simulink model "IDC_OS"  (R2023b)
settings: Solver=FixedStepAuto  StartTime=0.0  StopTime=9  FixedStep=sampleTime  RelTol=1e-3
values from neighbouring files (symbols this model uses):
  initialguess = robot.homeConfiguration    [IDC_OS.m]
  K_D = 0*eye(n_joints)    [IDC_OS.m]
  K_P = 0*eye(n_joints)    [IDC_OS.m]
  n_joints = 6    [IDC_OS.m]
  robot = loadrobot("universalUR5")    [IDC_OS.m]
  t0 = 0    [IDC_OS.m]
  t1 = 5    [IDC_OS.m]
  t2 = 10    [IDC_OS.m]
  t3 = 100    [IDC_OS.m]
  weights = transpose([0.1, 0.1, 0.1, 1, 1, 1])    [IDC_OS.m]
  x0_pose = trvec2tform([x0(1), x0(2), x0(3)]) * eul2tform([x0(4), x0(5), x0(6)])    [IDC_OS.m]
  xd = zeros(n_joints,1)    [IDC_OS.m]
undefined symbols (not defined in the file or in its folder): x1_pose, x2_pose
libraries: robotmaniplib x8
(part 1 of 2)
settings Model: Creator=Mikael  LastModifiedBy=Mikael

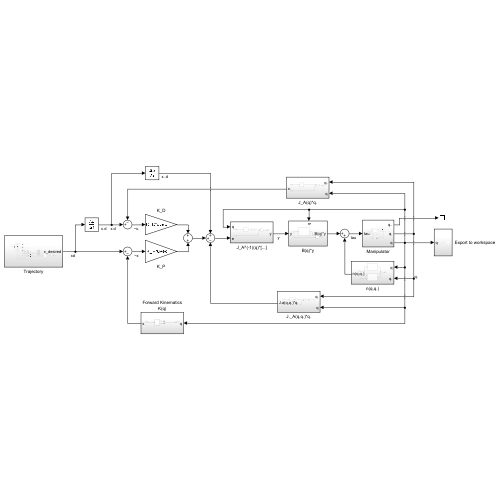
[thumbnail: Simulink's stored preview of the top-level diagram]
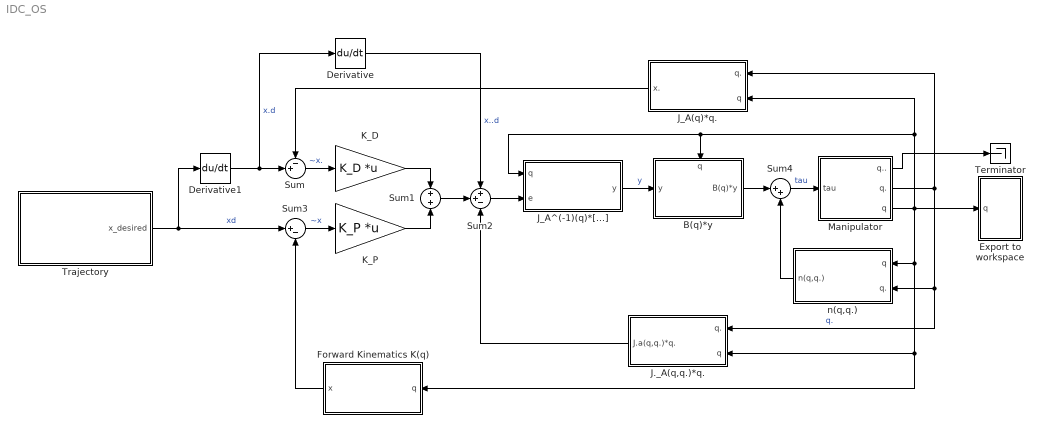
== system IDC_OS ==
  B(q)*y : Subsystem
      settings: PortSchema="{\"entries\":[{\"content\":{\"sides\":[{\"content\":{\"connectorIds\":[\"In1\"]},\"type\":\"ConnectorPlacement.EquallySpacedRectSide\",\"uuid\":\"33913df9-fd91-41b2-9bc7-1b3e33a51275\"},{\"content\":{\"connectorIds\":[\"Out1\"],\"side\":\"RIGHT\"},\"type\":\"ConnectorPlacement.EquallySpacedRectSide\",\"uuid\":\"b12fb46d-67b4-41c7-9bd3-75276d256d3b\"},{\"content\":{\"connectorIds\":[\"In2\"],\"side\":\"TOP\"},\"type\":\"ConnectorPlacement.EquallySpacedRectSide\",\"uuid\":\"ba102851-dd76-427a-8601-5d449287c868\"}]},\"type\":\"ConnectorPlacement.EquallySpacedConnector\",\"uuid\":\"a91f0b44-1456-4575-973a-6fc50432c507\"}],\"packageUris\":[\"http://schema.mathworks.com/mf0/Connector/R2020b\"],\"version\":\"1.0\"}"
  Derivative : Derivative
  Derivative1 : Derivative
  Export to workspace : Subsystem
  Forward Kinematics K(q) : Subsystem
  J._A(q,q.)*q. : Subsystem
  J_A(q)*q. : Subsystem
  J_A^(-1)(q)*[...] : Subsystem
  K_D : Gain  Gain=K_D  Multiplication=Matrix(K*u) (u vector)
  K_P : Gain  Gain=K_P  Multiplication=Matrix(K*u) (u vector)
  Manipulator : Subsystem
  Sum : Sum  Inputs=-+|
  Sum1 : Sum
  Sum2 : Sum  Inputs=++-
  Sum3 : Sum  Inputs=|+-
  Sum4 : Sum  Inputs=|++
  Terminator : Terminator
  Trajectory : Subsystem
  n(q,q.) : Subsystem
  wires:
  Manipulator/3(q) -> B(q)*y/2(q), J_A^(-1)(q)*[...]/1(q), J_A(q)*q./2(q), Export to workspace/1(q), J._A(q,q.)*q./2(q), Forward Kinematics K(q)/1(q), n(q,q.)/1(q)
  Manipulator/2(q.) -> J_A(q)*q./1(q.), J._A(q,q.)*q./1(q.), n(q,q.)/2(q.)  "q."
  Sum4/1 -> Manipulator/1(tau)  "tau"
  J_A(q)*q./1(x.) -> Sum/1
  Sum/1 -> K_D/1  "~x."
  Sum3/1 -> K_P/1  "~x"
  K_D/1 -> Sum1/1
  K_P/1 -> Sum1/2
  Sum2/1 -> J_A^(-1)(q)*[...]/2(e)
  Sum1/1 -> Sum2/2
  B(q)*y/1(B(q)*y) -> Sum4/1
  J_A^(-1)(q)*[...]/1(y) -> B(q)*y/1(y)  "y"
  n(q,q.)/1(n(q,q.)) -> Sum4/2
  J._A(q,q.)*q./1(J.a(q,q.)*q.) -> Sum2/3
  Forward Kinematics K(q)/1(x) -> Sum3/2
  Trajectory/1(x_desired) -> Sum3/1, Derivative1/1  "xd"
  Derivative1/1 -> Sum/2, Derivative/1  "x.d"
  Derivative/1 -> Sum2/1  "x..d"
  Manipulator/1(q..) -> Terminator/1

== system IDC_OS/B(q)*y ==
  y : Inport
  q : Inport  Port=2
  B(q) : robotmaniplib/Joint Space Mass Matrix  RigidBodyTree=robot  SimulateUsing=Code generation
  Matrix Multiply : Product  Multiplication=Matrix(*)
  B(q)*y : Outport
  wires:
  y/1 -> Matrix Multiply/2
  q/1 -> B(q)/1
  Matrix Multiply/1 -> B(q)*y/1
  B(q)/1 -> Matrix Multiply/1

== system IDC_OS/Export to workspace ==
  note: Export to workspace as:
      | - Array
      | - Save 2-D Signal as 3-D signal
      | (concatenated along the third dimension)
  q : Inport
  Signal Specification : SignalSpecification  Dimensions=[6,1]
  To Workspace2 : ToWorkspace  VariableName=q  SampleTime=-1
  wires:
  q/1 -> Signal Specification/1
  Signal Specification/1 -> To Workspace2/1

== system IDC_OS/Forward Kinematics K(q) ==
  q : Inport
  Direct Kinematics : Subsystem
  Mux : Mux  Inputs=2
  x : Outport
  wires:
  q/1 -> Direct Kinematics/1(q)
  Mux/1 -> x/1
  Direct Kinematics/1(position) -> Mux/1
  Direct Kinematics/2(orientation) -> Mux/2

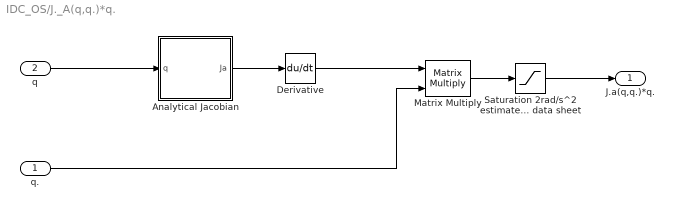
== system IDC_OS/J._A(q,q.)*q. ==
  q. : Inport
  q : Inport  Port=2
  Analytical Jacobian : Subsystem
  Derivative : Derivative
  Matrix Multiply : Product  Multiplication=Matrix(*)
  Saturation 2rad/s^2 estimated based on data sheet : Saturate  UpperLimit=2  LowerLimit=-2
  J.a(q,q.)*q. : Outport
  wires:
  q/1 -> Analytical Jacobian/1(q)
  q./1 -> Matrix Multiply/2
  Analytical Jacobian/1(Ja) -> Derivative/1
  Derivative/1 -> Matrix Multiply/1
  Matrix Multiply/1 -> Saturation 2rad/s^2 estimated based on data sheet/1
  Saturation 2rad/s^2 estimated based on data sheet/1 -> J.a(q,q.)*q./1

== system IDC_OS/J_A(q)*q. ==
  q. : Inport
  q : Inport  Port=2
  Analytical Jacobian : Subsystem
  Matrix Multiply : Product  Multiplication=Matrix(*)
  x. : Outport
  wires:
  q/1 -> Analytical Jacobian/1(q)
  q./1 -> Matrix Multiply/2
  Analytical Jacobian/1(Ja) -> Matrix Multiply/1
  Matrix Multiply/1 -> x./1

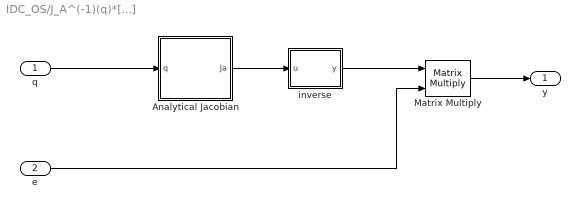
== system IDC_OS/J_A^(-1)(q)*[...] ==
  q : Inport
  e : Inport  Port=2
  Analytical Jacobian : Subsystem
  Matrix Multiply : Product  Multiplication=Matrix(*)
  inverse : MATLAB Function  TreatAsAtomicUnit=on
  y : Outport
  wires:
  q/1 -> Analytical Jacobian/1(q)
  e/1 -> Matrix Multiply/2
  inverse/1(y) -> Matrix Multiply/1
  Analytical Jacobian/1(Ja) -> inverse/1(u)
  Matrix Multiply/1 -> y/1

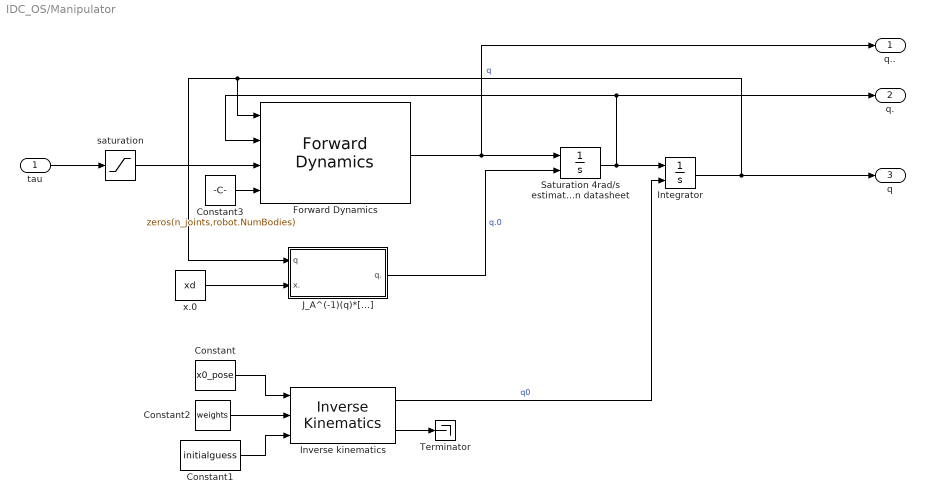
== system IDC_OS/Manipulator ==
  tau : Inport
  Constant : Constant  Value=x0_pose
  Constant1 : Constant  Value=initialguess
  Constant2 : Constant  Value=weights
  Constant3 : Constant  Value=zeros(n_joints,robot.NumBodies)
  Forward Dynamics : robotmaniplib/Forward Dynamics  RigidBodyTree=robot  SimulateUsing=Code generation
  Integrator : Integrator  InitialConditionSource=external
  Inverse kinematics : robotmaniplib/Inverse Kinematics  RigidBodyTree=robot  EndEffector=tool0  ShowInfo=on  SolverName=BFGS Gradient Projection  EnforceJointLimits=on  MaxIterations=1500  MaxTime=10  GradientTolerance=1e-7  SolutionTolerance=1e-6  StepTolerance=1e-14  ErrorChangeTolerance=1e-12  UseErrorDamping=on  DampingBias=0.0025  SimulateUsing=Code generation
  J_A^(-1)(q)*[...] : Subsystem
  Saturation 4rad/s estimated based on datasheet : Integrator  InitialConditionSource=external  LimitOutput=on  UpperSaturationLimit=4  LowerSaturationLimit=-4
  Terminator : Terminator
  saturation : Saturate  UpperLimit=inf  LowerLimit=-inf
  x.0 : Constant  Value=xd
  q.. : Outport
  q. : Outport  Port=2
  q : Outport  Port=3
  wires:
  Integrator/1 -> Forward Dynamics/1, J_A^(-1)(q)*[...]/1(q), q/1  "q"
  tau/1 -> saturation/1
  Inverse kinematics/1 -> Integrator/2  "q0"
  Constant/1 -> Inverse kinematics/1
  Constant2/1 -> Inverse kinematics/2
  Constant1/1 -> Inverse kinematics/3
  Saturation 4rad/s estimated based on datasheet/1 -> q./1, Forward Dynamics/2, Integrator/1
  saturation/1 -> Forward Dynamics/3
  Forward Dynamics/1 -> q../1, Saturation 4rad/s estimated based on datasheet/1
  J_A^(-1)(q)*[...]/1(q.) -> Saturation 4rad/s estimated based on datasheet/2  "q.0"
  x.0/1 -> J_A^(-1)(q)*[...]/2(x.)
  Constant3/1 -> Forward Dynamics/4
  Inverse kinematics/2 -> Terminator/1

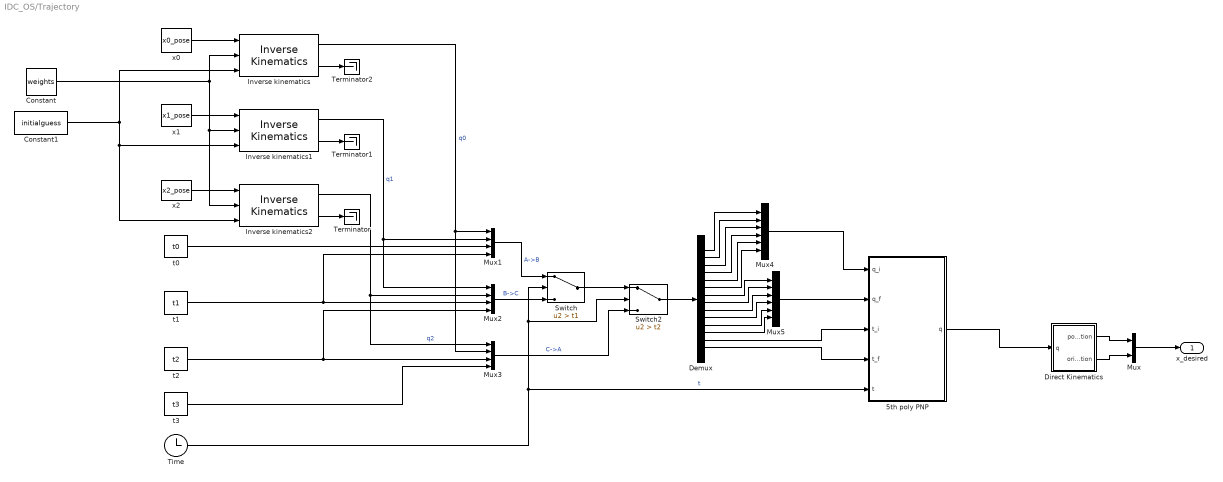
== system IDC_OS/Trajectory ==
  5th poly PNP : MATLAB Function  TreatAsAtomicUnit=on
  Constant : Constant  Value=weights
  Constant1 : Constant  Value=initialguess
  Demux : Demux  Outputs=14
  Direct Kinematics : Subsystem
  Inverse kinematics : robotmaniplib/Inverse Kinematics  RigidBodyTree=robot  EndEffector=tool0  ShowInfo=on  SolverName=BFGS Gradient Projection  EnforceJointLimits=on  MaxIterations=1500  MaxTime=10  GradientTolerance=1e-7  SolutionTolerance=1e-6  StepTolerance=1e-14  ErrorChangeTolerance=1e-12  UseErrorDamping=on  DampingBias=0.0025  SimulateUsing=Code generation
  Inverse kinematics1 : robotmaniplib/Inverse Kinematics  RigidBodyTree=robot  EndEffector=tool0  ShowInfo=on  SolverName=BFGS Gradient Projection  EnforceJointLimits=on  MaxIterations=1500  MaxTime=10  GradientTolerance=1e-7  SolutionTolerance=1e-6  StepTolerance=1e-14  ErrorChangeTolerance=1e-12  UseErrorDamping=on  DampingBias=0.0025  SimulateUsing=Code generation
  Inverse kinematics2 : robotmaniplib/Inverse Kinematics  RigidBodyTree=robot  EndEffector=tool0  ShowInfo=on  SolverName=BFGS Gradient Projection  EnforceJointLimits=on  MaxIterations=1500  MaxTime=10  GradientTolerance=1e-7  SolutionTolerance=1e-6  StepTolerance=1e-14  ErrorChangeTolerance=1e-12  UseErrorDamping=on  DampingBias=0.0025  SimulateUsing=Code generation
  Mux : Mux  Inputs=2
  Mux1 : Mux
  Mux2 : Mux
  Mux3 : Mux
  Mux4 : Mux  Inputs=6
  Mux5 : Mux  Inputs=6
  Switch : Switch  Criteria=u2 > Threshold  Threshold=t1  SaturateOnIntegerOverflow=off  InputSameDT=off
  Switch2 : Switch  Criteria=u2 > Threshold  Threshold=t2  SaturateOnIntegerOverflow=off  InputSameDT=off
  Terminator : Terminator
  Terminator1 : Terminator
  Terminator2 : Terminator
  Time : Clock
  t0 : Constant  Value=t0
  t1 : Constant  Value=t1
  t2 : Constant  Value=t2
  t3 : Constant  Value=t3
  x0 : Constant  Value=x0_pose
  x1 : Constant  Value=x1_pose
  x2 : Constant  Value=x2_pose
  x_desired : Outport
  wires:
  Direct Kinematics/1(position) -> Mux/1
  Direct Kinematics/2(orientation) -> Mux/2
  5th poly PNP/1(q) -> Direct Kinematics/1(q)
  Mux/1 -> x_desired/1
  x0/1 -> Inverse kinematics/1
  Time/1 -> Switch2/2, Switch/2, 5th poly PNP/5(t)  "t"
  Mux1/1 -> Switch/1  "A->B"
  Inverse kinematics/1 -> Mux3/2, Mux1/1  "q0"
  Inverse kinematics1/1 -> Mux2/1, Mux1/2  "q1"
  t0/1 -> Mux1/3
  t1/1 -> Mux2/3, Mux1/4
  Mux2/1 -> Switch/3  "B->C"
  Inverse kinematics2/1 -> Mux3/1, Mux2/2  "q2"
  t2/1 -> Mux3/3, Mux2/4
  t3/1 -> Mux3/4
  Switch/1 -> Switch2/1
  Switch2/1 -> Demux/1
  Mux3/1 -> Switch2/3  "C->A"
  Constant/1 -> Inverse kinematics2/2, Inverse kinematics1/2, Inverse kinematics/2
  x1/1 -> Inverse kinematics1/1
  x2/1 -> Inverse kinematics2/1
  Inverse kinematics2/2 -> Terminator/1
  Inverse kinematics1/2 -> Terminator1/1
  Inverse kinematics/2 -> Terminator2/1
  Constant1/1 -> Inverse kinematics2/3, Inverse kinematics1/3, Inverse kinematics/3
  Demux/1 -> Mux4/1
  Demux/2 -> Mux4/2
  Demux/3 -> Mux4/3
  Demux/4 -> Mux4/4
  Demux/5 -> Mux4/5
  Demux/6 -> Mux4/6
  Mux4/1 -> 5th poly PNP/1(q_i)
  Demux/7 -> Mux5/1
  Demux/8 -> Mux5/2
  Demux/9 -> Mux5/3
  Demux/10 -> Mux5/4
  Demux/11 -> Mux5/5
  Demux/12 -> Mux5/6
  Mux5/1 -> 5th poly PNP/2(q_f)
  Demux/13 -> 5th poly PNP/3(t_i)
  Demux/14 -> 5th poly PNP/4(t_f)

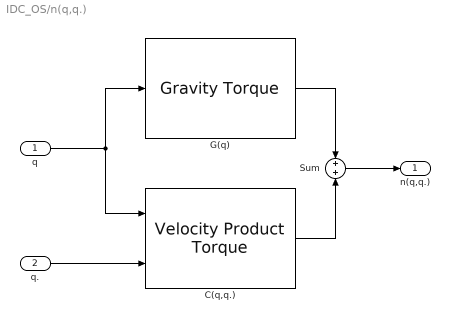
== system IDC_OS/n(q,q.) ==
  q : Inport
  q. : Inport  Port=2
  C(q,q.) : robotmaniplib/Velocity Product Torque  RigidBodyTree=robot  SimulateUsing=Code generation
  G(q) : robotmaniplib/Gravity Torque  RigidBodyTree=robot  SimulateUsing=Code generation
  Sum : Sum
  n(q,q.) : Outport
  wires:
  q./1 -> C(q,q.)/2
  q/1 -> C(q,q.)/1, G(q)/1
  G(q)/1 -> Sum/1
  C(q,q.)/1 -> Sum/2
  Sum/1 -> n(q,q.)/1

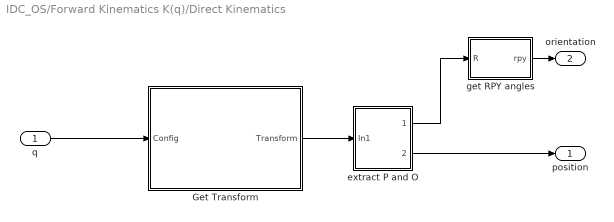
== system IDC_OS/Forward Kinematics K(q)/Direct Kinematics ==
  q : Inport
  Get Transform : Subsystem  mask(Get Transform){RigidBodyTree=robot, SourceBody=tool0, TargetBody=base, SimulateUsing=Code generation}
      mask prompts: RigidBodyTree "robotics:robotslmanip:blockmask:RigidBodyTreePrompt"; SourceBody "robotics:robotslmanip:blockmask:GetTransformSourceBodyPrompt"; TargetBody "robotics:robotslmanip:blockmask:GetTransformTargetBodyPrompt"; SimulateUsing "SystemBlock:MATLABSystem:SimulateUsing"
      mask help: robotics:robotslmanip:blockmask:GetTransformDescription
      mask init:
      | try
      |    [TreeStruct, NumBodies, sysName] = robotics.slmanip.internal.block.RBTAlgorithmBlockMasks.updateMaskWorkSpaceVariables(gcb, RigidBodyTree);
      |    robotics.slmanip.internal.block.RBTAlgorithmBlockMasks.updateBlockInputDimensions(gcb, TreeStruct, 'Config');
      | catch ME
      |    TreeStruct = [];  NumBodies = [];   sysName = '???';
      |    throw(ME);
      | end
      | SourceBodyArray = robotics.slmanip.internal.block.RBTAlgorithmBlockMasks.updateBodyWSVar(gcb, RigidBodyTree, 'SourceBody');
      | TargetBodyArray = robotics.slmanip.internal.block.RBTAlgorithmBlockMasks.updateBodyWSVar(gcb, RigidBodyTree, 'TargetBody');
      settings: LibrarySourceBlock=robotmaniplib/Get Transform
      mask Help: helpview(fullfile(docroot,'robotics','helptargets.map'), 'rstGetTransform');
      mask TypeOptions SimulateUsing: MATLAB System/SimulateUsing
      mask DialogControl RigidBodyTree Prompt: Rigid body tree:
      mask DialogControl SourceBody Prompt: Source body:
      mask DialogControl ListControl1 Prompt: Select body >>
      mask DialogControl ListControl1 Callback: robotics.slmanip.internal.block.RBTAlgorithmBlockMasks.updateMaskBodyList(gcb, 'SourceBody');
      mask DialogControl TargetBody Prompt: Target body:
      mask DialogControl ListControl2 Prompt: Select body >>
      mask DialogControl ListControl2 Callback: robotics.slmanip.internal.block.RBTAlgorithmBlockMasks.updateMaskBodyList(gcb, 'TargetBody');
      mask DialogControl SimulateUsing Prompt: Simulate using:
      mask DialogControl SimulateUsing Tooltip: SystemBlock:MATLABSystem:SimulateUsingDescription
      mask Display:
      | if (strcmp(sysName,'???'))
      | 	color('red');
      | else
      |     color('blue');
      | end
      | text(0.99, 0.99, sysName, 'horizontalAlignment', 'right', 'verticalAlignment','top');
      | 
      | color('black')
      | SourceText = ['Source: ' get_param(gcb,'SourceBody')];
      | TargetText = ['Target: ' get_param(gcb,'TargetBody')];
      | DescText = [SourceText newline TargetText];
      | text(0.5, 0.05, DescText, 'horizontalAlignment', 'center','verticalAlignment','bottom');
      | 
      | port_label('input', 1, 'Config')
      | port_label('output', 1, 'Transform')
  extract P and O : Subsystem
  get RPY angles : MATLAB Function  TreatAsAtomicUnit=on
  position : Outport
  orientation : Outport  Port=2
  wires:
  get RPY angles/1(rpy) -> orientation/1
  extract P and O/1(orientation) -> get RPY angles/1(R)
  extract P and O/2(position) -> position/1
  Get Transform/1(Transform) -> extract P and O/1(In1)
  q/1 -> Get Transform/1(Config)

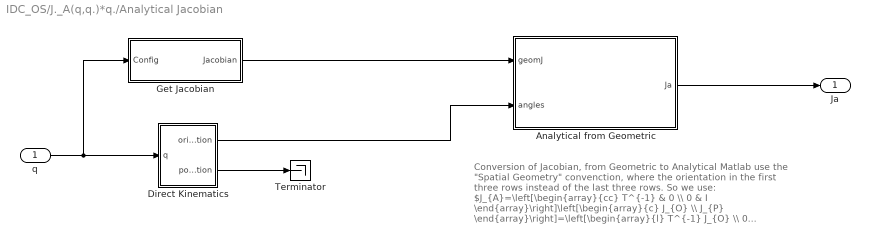
== system IDC_OS/J._A(q,q.)*q./Analytical Jacobian ==
  note: Conversion of Jacobian, from Geometric to Analytical
      |
      | Matlab use the "Spatial Geometry" convenction, where the orientation in the first three rows instead of the last three rows. So we use:
      |
      | $J_{A}=\left[\begin{array}{cc} T^{-1} & 0 \\ 0 & I \end{array}\right]\left[\begin{array}{c} J_{O} \\ J_{P} \end{array}\right]=\left[\begin{array}{l} T^{-1} J_{O} \\ 0 \end{array}\right]+\left[\begin{array}{c} 0\\ J_{P} \end{array}\right] \quad \text {if } \,\, J=\left[\begin{array}{l} J_{O} \\ J_{P} \end{array}\right]$
      |
      | If orientation is in the last three rows (as in most of the text books) we would use instead:
      |
      | $J_{A}=\left[\begin{array}{cc} I & 0 \\ 0 & T^{-1} \end{array}\right]\left[\begin{array}{c} J_{P} \\ J_{O} \end{array}\right]=\left[\begin{array}{l} J_{P} \\ 0 \end{array}\right]+\left[\begin{array}{c} 0\\ T^{-1} J_{O} \end{array}\right] \quad \text { if } \,\, J=\left[\begin{array}{l} J_{P} \\ J_{O} \end{array}\right]$
  q : Inport
  Analytical from Geometric : MATLAB Function  TreatAsAtomicUnit=on
  Direct Kinematics : Subsystem
  Get Jacobian : Subsystem  mask(Get Jacobian){RigidBodyTree=robot, EndEffector=tool0, SimulateUsing=Code generation}
      mask prompts: RigidBodyTree "robotics:robotslmanip:blockmask:RigidBodyTreePrompt"; EndEffector "robotics:robotslmanip:blockmask:EndEffectorPrompt"; SimulateUsing "SystemBlock:MATLABSystem:SimulateUsing"
      mask help: robotics:robotslmanip:blockmask:GetJacobianDescription
      mask init:
      | try
      |    [TreeStruct, NumBodies, sysName] = robotics.slmanip.internal.block.RBTAlgorithmBlockMasks.updateMaskWorkSpaceVariables(gcb, RigidBodyTree);
      |    robotics.slmanip.internal.block.RBTAlgorithmBlockMasks.updateBlockInputDimensions(gcb, TreeStruct, 'Config');
      | catch ME
      |    TreeStruct = [];  NumBodies = [];   sysName = '???';
      |    throw(ME);
      | end
      | EndEffectorArray = robotics.slmanip.internal.block.RBTAlgorithmBlockMasks.updateBodyWSVar(gcb, RigidBodyTree, 'EndEffector');
      settings: LibrarySourceBlock=robotmaniplib/Get Jacobian
      mask Help: helpview(fullfile(docroot,'robotics','helptargets.map'), 'rstGetJacobian');
      mask TypeOptions SimulateUsing: MATLAB System/SimulateUsing
      mask DialogControl RigidBodyTree Prompt: Rigid body tree:
      mask DialogControl EndEffector Prompt: End effector:
      mask DialogControl ListControl Prompt: robotics:robotslmanip:blockmask:SelectBodyButtonPrompt
      mask DialogControl ListControl Callback: robotics.slmanip.internal.block.RBTAlgorithmBlockMasks.updateMaskBodyList(gcb, 'EndEffector');
      mask DialogControl SimulateUsing Prompt: Simulate using:
      mask DialogControl SimulateUsing Tooltip: SystemBlock:MATLABSystem:SimulateUsingDescription
      mask Display:
      | if (strcmp(sysName,'???'))
      | 	color('red');
      | else
      |     color('blue');
      | end
      | text(0.99, 0.99, sysName, 'horizontalAlignment', 'right', 'verticalAlignment','top');
      | 
      | color('black');
      | DescText = ['EE: ' get_param(gcb,'EndEffector')];
      | text(0.5, 0.05, DescText, 'horizontalAlignment', 'center', 'verticalAlignment','bottom');
      | 
      | port_label('input', 1, 'Config')
      | port_label('output', 1, 'Jacobian')
  Terminator : Terminator
  Ja : Outport
  wires:
  Direct Kinematics/1(orientation) -> Analytical from Geometric/2(angles)
  Direct Kinematics/2(position) -> Terminator/1
  Analytical from Geometric/1(Ja) -> Ja/1
  Get Jacobian/1(Jacobian) -> Analytical from Geometric/1(geomJ)
  q/1 -> Get Jacobian/1(Config), Direct Kinematics/1(q)

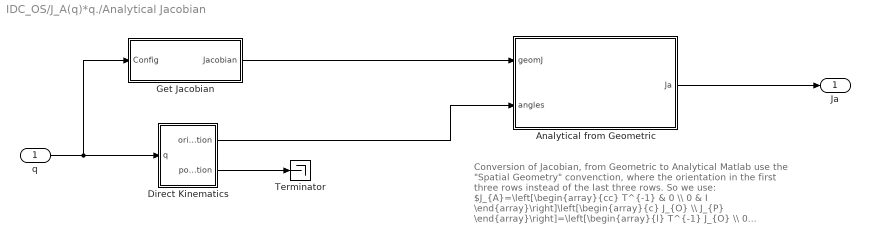
== system IDC_OS/J_A(q)*q./Analytical Jacobian ==
  note: Conversion of Jacobian, from Geometric to Analytical
      |
      | Matlab use the "Spatial Geometry" convenction, where the orientation in the first three rows instead of the last three rows. So we use:
      |
      | $J_{A}=\left[\begin{array}{cc} T^{-1} & 0 \\ 0 & I \end{array}\right]\left[\begin{array}{c} J_{O} \\ J_{P} \end{array}\right]=\left[\begin{array}{l} T^{-1} J_{O} \\ 0 \end{array}\right]+\left[\begin{array}{c} 0\\ J_{P} \end{array}\right] \quad \text {if } \,\, J=\left[\begin{array}{l} J_{O} \\ J_{P} \end{array}\right]$
      |
      | If orientation is in the last three rows (as in most of the text books) we would use instead:
      |
      | $J_{A}=\left[\begin{array}{cc} I & 0 \\ 0 & T^{-1} \end{array}\right]\left[\begin{array}{c} J_{P} \\ J_{O} \end{array}\right]=\left[\begin{array}{l} J_{P} \\ 0 \end{array}\right]+\left[\begin{array}{c} 0\\ T^{-1} J_{O} \end{array}\right] \quad \text { if } \,\, J=\left[\begin{array}{l} J_{P} \\ J_{O} \end{array}\right]$
  q : Inport
  Analytical from Geometric : MATLAB Function  TreatAsAtomicUnit=on
  Direct Kinematics : Subsystem
  Get Jacobian : Subsystem  mask(Get Jacobian){RigidBodyTree=robot, EndEffector=tool0, SimulateUsing=Code generation}
      mask prompts: RigidBodyTree "robotics:robotslmanip:blockmask:RigidBodyTreePrompt"; EndEffector "robotics:robotslmanip:blockmask:EndEffectorPrompt"; SimulateUsing "SystemBlock:MATLABSystem:SimulateUsing"
      mask help: robotics:robotslmanip:blockmask:GetJacobianDescription
      mask init: same as IDC_OS/J._A(q,q.)*q./Analytical Jacobian/Get Jacobian
      settings: LibrarySourceBlock=robotmaniplib/Get Jacobian
      mask Help: helpview(fullfile(docroot,'robotics','helptargets.map'), 'rstGetJacobian');
      mask TypeOptions SimulateUsing: MATLAB System/SimulateUsing
      mask DialogControl RigidBodyTree Prompt: Rigid body tree:
      mask DialogControl EndEffector Prompt: End effector:
      mask DialogControl ListControl Prompt: robotics:robotslmanip:blockmask:SelectBodyButtonPrompt
      mask DialogControl ListControl Callback: robotics.slmanip.internal.block.RBTAlgorithmBlockMasks.updateMaskBodyList(gcb, 'EndEffector');
      mask DialogControl SimulateUsing Prompt: Simulate using:
      mask DialogControl SimulateUsing Tooltip: SystemBlock:MATLABSystem:SimulateUsingDescription
      mask Display:
      | if (strcmp(sysName,'???'))
      | 	color('red');
      | else
      |     color('blue');
      | end
      | text(0.99, 0.99, sysName, 'horizontalAlignment', 'right', 'verticalAlignment','top');
      | 
      | color('black');
      | DescText = ['EE: ' get_param(gcb,'EndEffector')];
      | text(0.5, 0.05, DescText, 'horizontalAlignment', 'center', 'verticalAlignment','bottom');
      | 
      | port_label('input', 1, 'Config')
      | port_label('output', 1, 'Jacobian')
  Terminator : Terminator
  Ja : Outport
  wires:
  Direct Kinematics/1(orientation) -> Analytical from Geometric/2(angles)
  Direct Kinematics/2(position) -> Terminator/1
  Analytical from Geometric/1(Ja) -> Ja/1
  Get Jacobian/1(Jacobian) -> Analytical from Geometric/1(geomJ)
  q/1 -> Get Jacobian/1(Config), Direct Kinematics/1(q)

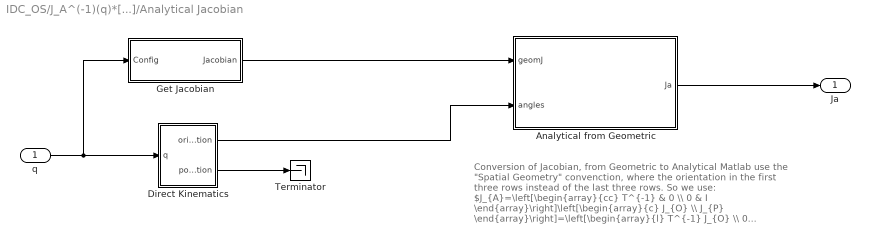
== system IDC_OS/J_A^(-1)(q)*[...]/Analytical Jacobian ==
  note: Conversion of Jacobian, from Geometric to Analytical
      |
      | Matlab use the "Spatial Geometry" convenction, where the orientation in the first three rows instead of the last three rows. So we use:
      |
      | $J_{A}=\left[\begin{array}{cc} T^{-1} & 0 \\ 0 & I \end{array}\right]\left[\begin{array}{c} J_{O} \\ J_{P} \end{array}\right]=\left[\begin{array}{l} T^{-1} J_{O} \\ 0 \end{array}\right]+\left[\begin{array}{c} 0\\ J_{P} \end{array}\right] \quad \text {if } \,\, J=\left[\begin{array}{l} J_{O} \\ J_{P} \end{array}\right]$
      |
      | If orientation is in the last three rows (as in most of the text books) we would use instead:
      |
      | $J_{A}=\left[\begin{array}{cc} I & 0 \\ 0 & T^{-1} \end{array}\right]\left[\begin{array}{c} J_{P} \\ J_{O} \end{array}\right]=\left[\begin{array}{l} J_{P} \\ 0 \end{array}\right]+\left[\begin{array}{c} 0\\ T^{-1} J_{O} \end{array}\right] \quad \text { if } \,\, J=\left[\begin{array}{l} J_{P} \\ J_{O} \end{array}\right]$
  q : Inport
  Analytical from Geometric : MATLAB Function  TreatAsAtomicUnit=on
  Direct Kinematics : Subsystem
  Get Jacobian : Subsystem  mask(Get Jacobian){RigidBodyTree=robot, EndEffector=tool0, SimulateUsing=Code generation}
      mask prompts: RigidBodyTree "robotics:robotslmanip:blockmask:RigidBodyTreePrompt"; EndEffector "robotics:robotslmanip:blockmask:EndEffectorPrompt"; SimulateUsing "SystemBlock:MATLABSystem:SimulateUsing"
      mask help: robotics:robotslmanip:blockmask:GetJacobianDescription
      mask init: same as IDC_OS/J._A(q,q.)*q./Analytical Jacobian/Get Jacobian
      settings: LibrarySourceBlock=robotmaniplib/Get Jacobian
      mask Help: helpview(fullfile(docroot,'robotics','helptargets.map'), 'rstGetJacobian');
      mask TypeOptions SimulateUsing: MATLAB System/SimulateUsing
      mask DialogControl RigidBodyTree Prompt: Rigid body tree:
      mask DialogControl EndEffector Prompt: End effector:
      mask DialogControl ListControl Prompt: robotics:robotslmanip:blockmask:SelectBodyButtonPrompt
      mask DialogControl ListControl Callback: robotics.slmanip.internal.block.RBTAlgorithmBlockMasks.updateMaskBodyList(gcb, 'EndEffector');
      mask DialogControl SimulateUsing Prompt: Simulate using:
      mask DialogControl SimulateUsing Tooltip: SystemBlock:MATLABSystem:SimulateUsingDescription
      mask Display:
      | if (strcmp(sysName,'???'))
      | 	color('red');
      | else
      |     color('blue');
      | end
      | text(0.99, 0.99, sysName, 'horizontalAlignment', 'right', 'verticalAlignment','top');
      | 
      | color('black');
      | DescText = ['EE: ' get_param(gcb,'EndEffector')];
      | text(0.5, 0.05, DescText, 'horizontalAlignment', 'center', 'verticalAlignment','bottom');
      | 
      | port_label('input', 1, 'Config')
      | port_label('output', 1, 'Jacobian')
  Terminator : Terminator
  Ja : Outport
  wires:
  Direct Kinematics/1(orientation) -> Analytical from Geometric/2(angles)
  Direct Kinematics/2(position) -> Terminator/1
  Analytical from Geometric/1(Ja) -> Ja/1
  Get Jacobian/1(Jacobian) -> Analytical from Geometric/1(geomJ)
  q/1 -> Get Jacobian/1(Config), Direct Kinematics/1(q)

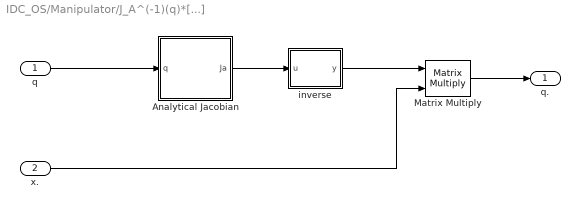
== system IDC_OS/Manipulator/J_A^(-1)(q)*[...] ==
  q : Inport
  x. : Inport  Port=2
  Analytical Jacobian : Subsystem
  Matrix Multiply : Product  Multiplication=Matrix(*)
  inverse : MATLAB Function  TreatAsAtomicUnit=on
  q. : Outport
  wires:
  q/1 -> Analytical Jacobian/1(q)
  x./1 -> Matrix Multiply/2
  inverse/1(y) -> Matrix Multiply/1
  Analytical Jacobian/1(Ja) -> inverse/1(u)
  Matrix Multiply/1 -> q./1

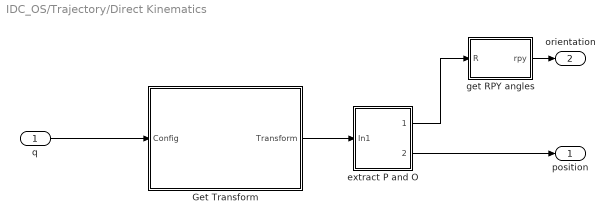
== system IDC_OS/Trajectory/Direct Kinematics ==
  q : Inport
  Get Transform : Subsystem  mask(Get Transform){RigidBodyTree=robot, SourceBody=tool0, TargetBody=base, SimulateUsing=Code generation}
      mask prompts: RigidBodyTree "robotics:robotslmanip:blockmask:RigidBodyTreePrompt"; SourceBody "robotics:robotslmanip:blockmask:GetTransformSourceBodyPrompt"; TargetBody "robotics:robotslmanip:blockmask:GetTransformTargetBodyPrompt"; SimulateUsing "SystemBlock:MATLABSystem:SimulateUsing"
      mask help: robotics:robotslmanip:blockmask:GetTransformDescription
      mask init: same as IDC_OS/Forward Kinematics K(q)/Direct Kinematics/Get Transform
      settings: LibrarySourceBlock=robotmaniplib/Get Transform
      mask Help: helpview(fullfile(docroot,'robotics','helptargets.map'), 'rstGetTransform');
      mask TypeOptions SimulateUsing: MATLAB System/SimulateUsing
      mask DialogControl RigidBodyTree Prompt: Rigid body tree:
      mask DialogControl SourceBody Prompt: Source body:
      mask DialogControl ListControl1 Prompt: Select body >>
      mask DialogControl ListControl1 Callback: robotics.slmanip.internal.block.RBTAlgorithmBlockMasks.updateMaskBodyList(gcb, 'SourceBody');
      mask DialogControl TargetBody Prompt: Target body:
      mask DialogControl ListControl2 Prompt: Select body >>
      mask DialogControl ListControl2 Callback: robotics.slmanip.internal.block.RBTAlgorithmBlockMasks.updateMaskBodyList(gcb, 'TargetBody');
      mask DialogControl SimulateUsing Prompt: Simulate using:
      mask DialogControl SimulateUsing Tooltip: SystemBlock:MATLABSystem:SimulateUsingDescription
      mask Display:
      | if (strcmp(sysName,'???'))
      | 	color('red');
      | else
      |     color('blue');
      | end
      | text(0.99, 0.99, sysName, 'horizontalAlignment', 'right', 'verticalAlignment','top');
      | 
      | color('black')
      | SourceText = ['Source: ' get_param(gcb,'SourceBody')];
      | TargetText = ['Target: ' get_param(gcb,'TargetBody')];
      | DescText = [SourceText newline TargetText];
      | text(0.5, 0.05, DescText, 'horizontalAlignment', 'center','verticalAlignment','bottom');
      | 
      | port_label('input', 1, 'Config')
      | port_label('output', 1, 'Transform')
  extract P and O : Subsystem
  get RPY angles : MATLAB Function  TreatAsAtomicUnit=on
  position : Outport
  orientation : Outport  Port=2
  wires:
  get RPY angles/1(rpy) -> orientation/1
  extract P and O/1(orientation) -> get RPY angles/1(R)
  extract P and O/2(position) -> position/1
  Get Transform/1(Transform) -> extract P and O/1(In1)
  q/1 -> Get Transform/1(Config)

== system IDC_OS/Forward Kinematics K(q)/Direct Kinematics/Get Transform ==
  Config : Inport  PortDimensions=6
  MATLAB System : MATLABSystem  System=robotics.slmanip.internal.block.GetTransformBlock  TreeStruct=TreeStruct  SourceBodyName=SourceBody  TargetBodyName=TargetBody  SimulateUsing=Code generation
      mask Type: robotics.slmanip.internal.block.GetTransformBlock
      mask Display:
      | disp('GetTransformBlock');
      | port_label('input',1,'q');
      | port_label('output',1,'tform');
  Transform : Outport  VectorParamsAs1DForOutWhenUnconnected=off
  wires:
  MATLAB System/1 -> Transform/1
  Config/1 -> MATLAB System/1

== system IDC_OS/Forward Kinematics K(q)/Direct Kinematics/extract P and O ==
  In1 : Inport
  Orientation : MATLABFcn  MATLABFcn=tform2rotm  Output1D=off
  Position : MATLABFcn  MATLABFcn=tform2trvec
  orientation : Outport
  position : Outport  Port=2
  wires:
  Orientation/1 -> orientation/1
  In1/1 -> Position/1, Orientation/1
  Position/1 -> position/1

== system IDC_OS/J._A(q,q.)*q./Analytical Jacobian/Direct Kinematics ==
  q : Inport
  Get Transform : Subsystem  mask(Get Transform){RigidBodyTree=robot, SourceBody=tool0, TargetBody=base, SimulateUsing=Code generation}
      mask prompts: RigidBodyTree "robotics:robotslmanip:blockmask:RigidBodyTreePrompt"; SourceBody "robotics:robotslmanip:blockmask:GetTransformSourceBodyPrompt"; TargetBody "robotics:robotslmanip:blockmask:GetTransformTargetBodyPrompt"; SimulateUsing "SystemBlock:MATLABSystem:SimulateUsing"
      mask help: robotics:robotslmanip:blockmask:GetTransformDescription
      mask init: same as IDC_OS/Forward Kinematics K(q)/Direct Kinematics/Get Transform
      settings: LibrarySourceBlock=robotmaniplib/Get Transform
      mask Help: helpview(fullfile(docroot,'robotics','helptargets.map'), 'rstGetTransform');
      mask TypeOptions SimulateUsing: MATLAB System/SimulateUsing
      mask DialogControl RigidBodyTree Prompt: Rigid body tree:
      mask DialogControl SourceBody Prompt: Source body:
      mask DialogControl ListControl1 Prompt: Select body >>
      mask DialogControl ListControl1 Callback: robotics.slmanip.internal.block.RBTAlgorithmBlockMasks.updateMaskBodyList(gcb, 'SourceBody');
      mask DialogControl TargetBody Prompt: Target body:
      mask DialogControl ListControl2 Prompt: Select body >>
      mask DialogControl ListControl2 Callback: robotics.slmanip.internal.block.RBTAlgorithmBlockMasks.updateMaskBodyList(gcb, 'TargetBody');
      mask DialogControl SimulateUsing Prompt: Simulate using:
      mask DialogControl SimulateUsing Tooltip: SystemBlock:MATLABSystem:SimulateUsingDescription
      mask Display:
      | if (strcmp(sysName,'???'))
      | 	color('red');
      | else
      |     color('blue');
      | end
      | text(0.99, 0.99, sysName, 'horizontalAlignment', 'right', 'verticalAlignment','top');
      | 
      | color('black')
      | SourceText = ['Source: ' get_param(gcb,'SourceBody')];
      | TargetText = ['Target: ' get_param(gcb,'TargetBody')];
      | DescText = [SourceText newline TargetText];
      | text(0.5, 0.05, DescText, 'horizontalAlignment', 'center','verticalAlignment','bottom');
      | 
      | port_label('input', 1, 'Config')
      | port_label('output', 1, 'Transform')
  extract P and O : Subsystem
  get RPY angles : MATLAB Function  TreatAsAtomicUnit=on
  orientation : Outport
  position : Outport  Port=2
  wires:
  get RPY angles/1(rpy) -> orientation/1
  extract P and O/1(orientation) -> get RPY angles/1(R)
  extract P and O/2(position) -> position/1
  Get Transform/1(Transform) -> extract P and O/1(In1)
  q/1 -> Get Transform/1(Config)

== system IDC_OS/J._A(q,q.)*q./Analytical Jacobian/Get Jacobian ==
  Config : Inport  PortDimensions=6
  MATLAB System : MATLABSystem  System=robotics.slmanip.internal.block.GetJacobianBlock  TreeStruct=TreeStruct  EEBodyName=EndEffector  SimulateUsing=Code generation
      mask Type: robotics.slmanip.internal.block.GetJacobianBlock
      mask Display:
      | disp('GetJacobianBlock');
      | port_label('input',1,'q');
      | port_label('output',1,'jacobianMat');
  Jacobian : Outport  VectorParamsAs1DForOutWhenUnconnected=off
  wires:
  MATLAB System/1 -> Jacobian/1
  Config/1 -> MATLAB System/1

== system IDC_OS/J_A(q)*q./Analytical Jacobian/Direct Kinematics ==
  q : Inport
  Get Transform : Subsystem  mask(Get Transform){RigidBodyTree=robot, SourceBody=tool0, TargetBody=base, SimulateUsing=Code generation}
      mask prompts: RigidBodyTree "robotics:robotslmanip:blockmask:RigidBodyTreePrompt"; SourceBody "robotics:robotslmanip:blockmask:GetTransformSourceBodyPrompt"; TargetBody "robotics:robotslmanip:blockmask:GetTransformTargetBodyPrompt"; SimulateUsing "SystemBlock:MATLABSystem:SimulateUsing"
      mask help: robotics:robotslmanip:blockmask:GetTransformDescription
      mask init: same as IDC_OS/Forward Kinematics K(q)/Direct Kinematics/Get Transform
      settings: LibrarySourceBlock=robotmaniplib/Get Transform
      mask Help: helpview(fullfile(docroot,'robotics','helptargets.map'), 'rstGetTransform');
      mask TypeOptions SimulateUsing: MATLAB System/SimulateUsing
      mask DialogControl RigidBodyTree Prompt: Rigid body tree:
      mask DialogControl SourceBody Prompt: Source body:
      mask DialogControl ListControl1 Prompt: Select body >>
      mask DialogControl ListControl1 Callback: robotics.slmanip.internal.block.RBTAlgorithmBlockMasks.updateMaskBodyList(gcb, 'SourceBody');
      mask DialogControl TargetBody Prompt: Target body:
      mask DialogControl ListControl2 Prompt: Select body >>
      mask DialogControl ListControl2 Callback: robotics.slmanip.internal.block.RBTAlgorithmBlockMasks.updateMaskBodyList(gcb, 'TargetBody');
      mask DialogControl SimulateUsing Prompt: Simulate using:
      mask DialogControl SimulateUsing Tooltip: SystemBlock:MATLABSystem:SimulateUsingDescription
      mask Display:
      | if (strcmp(sysName,'???'))
      | 	color('red');
      | else
      |     color('blue');
      | end
      | text(0.99, 0.99, sysName, 'horizontalAlignment', 'right', 'verticalAlignment','top');
      | 
      | color('black')
      | SourceText = ['Source: ' get_param(gcb,'SourceBody')];
      | TargetText = ['Target: ' get_param(gcb,'TargetBody')];
      | DescText = [SourceText newline TargetText];
      | text(0.5, 0.05, DescText, 'horizontalAlignment', 'center','verticalAlignment','bottom');
      | 
      | port_label('input', 1, 'Config')
      | port_label('output', 1, 'Transform')
  extract P and O : Subsystem
  get RPY angles : MATLAB Function  TreatAsAtomicUnit=on
  orientation : Outport
  position : Outport  Port=2
  wires:
  get RPY angles/1(rpy) -> orientation/1
  extract P and O/1(orientation) -> get RPY angles/1(R)
  extract P and O/2(position) -> position/1
  Get Transform/1(Transform) -> extract P and O/1(In1)
  q/1 -> Get Transform/1(Config)

== system IDC_OS/J_A(q)*q./Analytical Jacobian/Get Jacobian ==
  Config : Inport  PortDimensions=6
  MATLAB System : MATLABSystem  System=robotics.slmanip.internal.block.GetJacobianBlock  TreeStruct=TreeStruct  EEBodyName=EndEffector  SimulateUsing=Code generation
      mask Type: robotics.slmanip.internal.block.GetJacobianBlock
      mask Display:
      | disp('GetJacobianBlock');
      | port_label('input',1,'q');
      | port_label('output',1,'jacobianMat');
  Jacobian : Outport  VectorParamsAs1DForOutWhenUnconnected=off
  wires:
  MATLAB System/1 -> Jacobian/1
  Config/1 -> MATLAB System/1

== system IDC_OS/J_A^(-1)(q)*[...]/Analytical Jacobian/Direct Kinematics ==
  q : Inport
  Get Transform : Subsystem  mask(Get Transform){RigidBodyTree=robot, SourceBody=tool0, TargetBody=base, SimulateUsing=Code generation}
      mask prompts: RigidBodyTree "robotics:robotslmanip:blockmask:RigidBodyTreePrompt"; SourceBody "robotics:robotslmanip:blockmask:GetTransformSourceBodyPrompt"; TargetBody "robotics:robotslmanip:blockmask:GetTransformTargetBodyPrompt"; SimulateUsing "SystemBlock:MATLABSystem:SimulateUsing"
      mask help: robotics:robotslmanip:blockmask:GetTransformDescription
      mask init: same as IDC_OS/Forward Kinematics K(q)/Direct Kinematics/Get Transform
      settings: LibrarySourceBlock=robotmaniplib/Get Transform
      mask Help: helpview(fullfile(docroot,'robotics','helptargets.map'), 'rstGetTransform');
      mask TypeOptions SimulateUsing: MATLAB System/SimulateUsing
      mask DialogControl RigidBodyTree Prompt: Rigid body tree:
      mask DialogControl SourceBody Prompt: Source body:
      mask DialogControl ListControl1 Prompt: Select body >>
      mask DialogControl ListControl1 Callback: robotics.slmanip.internal.block.RBTAlgorithmBlockMasks.updateMaskBodyList(gcb, 'SourceBody');
      mask DialogControl TargetBody Prompt: Target body:
      mask DialogControl ListControl2 Prompt: Select body >>
      mask DialogControl ListControl2 Callback: robotics.slmanip.internal.block.RBTAlgorithmBlockMasks.updateMaskBodyList(gcb, 'TargetBody');
      mask DialogControl SimulateUsing Prompt: Simulate using:
      mask DialogControl SimulateUsing Tooltip: SystemBlock:MATLABSystem:SimulateUsingDescription
      mask Display:
      | if (strcmp(sysName,'???'))
      | 	color('red');
      | else
      |     color('blue');
      | end
      | text(0.99, 0.99, sysName, 'horizontalAlignment', 'right', 'verticalAlignment','top');
      | 
      | color('black')
      | SourceText = ['Source: ' get_param(gcb,'SourceBody')];
      | TargetText = ['Target: ' get_param(gcb,'TargetBody')];
      | DescText = [SourceText newline TargetText];
      | text(0.5, 0.05, DescText, 'horizontalAlignment', 'center','verticalAlignment','bottom');
      | 
      | port_label('input', 1, 'Config')
      | port_label('output', 1, 'Transform')
  extract P and O : Subsystem
  get RPY angles : MATLAB Function  TreatAsAtomicUnit=on
  orientation : Outport
  position : Outport  Port=2
  wires:
  get RPY angles/1(rpy) -> orientation/1
  extract P and O/1(orientation) -> get RPY angles/1(R)
  extract P and O/2(position) -> position/1
  Get Transform/1(Transform) -> extract P and O/1(In1)
  q/1 -> Get Transform/1(Config)

== system IDC_OS/J_A^(-1)(q)*[...]/Analytical Jacobian/Get Jacobian ==
  Config : Inport  PortDimensions=6
  MATLAB System : MATLABSystem  System=robotics.slmanip.internal.block.GetJacobianBlock  TreeStruct=TreeStruct  EEBodyName=EndEffector  SimulateUsing=Code generation
      mask Type: robotics.slmanip.internal.block.GetJacobianBlock
      mask Display:
      | disp('GetJacobianBlock');
      | port_label('input',1,'q');
      | port_label('output',1,'jacobianMat');
  Jacobian : Outport  VectorParamsAs1DForOutWhenUnconnected=off
  wires:
  MATLAB System/1 -> Jacobian/1
  Config/1 -> MATLAB System/1

== system IDC_OS/Manipulator/J_A^(-1)(q)*[...]/Analytical Jacobian ==
  note: Conversion of Jacobian, from Geometric to Analytical
      |
      | Matlab use the "Spatial Geometry" convenction, where the orientation in the first three rows instead of the last three rows. So we use:
      |
      | $J_{A}=\left[\begin{array}{cc} T^{-1} & 0 \\ 0 & I \end{array}\right]\left[\begin{array}{c} J_{O} \\ J_{P} \end{array}\right]=\left[\begin{array}{l} T^{-1} J_{O} \\ 0 \end{array}\right]+\left[\begin{array}{c} 0\\ J_{P} \end{array}\right] \quad \text {if } \,\, J=\left[\begin{array}{l} J_{O} \\ J_{P} \end{array}\right]$
      |
      | If orientation is in the last three rows (as in most of the text books) we would use instead:
      |
      | $J_{A}=\left[\begin{array}{cc} I & 0 \\ 0 & T^{-1} \end{array}\right]\left[\begin{array}{c} J_{P} \\ J_{O} \end{array}\right]=\left[\begin{array}{l} J_{P} \\ 0 \end{array}\right]+\left[\begin{array}{c} 0\\ T^{-1} J_{O} \end{array}\right] \quad \text { if } \,\, J=\left[\begin{array}{l} J_{P} \\ J_{O} \end{array}\right]$
  q : Inport
  Analytical from Geometric : MATLAB Function  TreatAsAtomicUnit=on
  Direct Kinematics : Subsystem
  Get Jacobian : Subsystem  mask(Get Jacobian){RigidBodyTree=robot, EndEffector=tool0, SimulateUsing=Code generation}
      mask prompts: RigidBodyTree "robotics:robotslmanip:blockmask:RigidBodyTreePrompt"; EndEffector "robotics:robotslmanip:blockmask:EndEffectorPrompt"; SimulateUsing "SystemBlock:MATLABSystem:SimulateUsing"
      mask help: robotics:robotslmanip:blockmask:GetJacobianDescription
      mask init: same as IDC_OS/J._A(q,q.)*q./Analytical Jacobian/Get Jacobian
      settings: LibrarySourceBlock=robotmaniplib/Get Jacobian
      mask Help: helpview(fullfile(docroot,'robotics','helptargets.map'), 'rstGetJacobian');
      mask TypeOptions SimulateUsing: MATLAB System/SimulateUsing
      mask DialogControl RigidBodyTree Prompt: Rigid body tree:
      mask DialogControl EndEffector Prompt: End effector:
      mask DialogControl ListControl Prompt: robotics:robotslmanip:blockmask:SelectBodyButtonPrompt
      mask DialogControl ListControl Callback: robotics.slmanip.internal.block.RBTAlgorithmBlockMasks.updateMaskBodyList(gcb, 'EndEffector');
      mask DialogControl SimulateUsing Prompt: Simulate using:
      mask DialogControl SimulateUsing Tooltip: SystemBlock:MATLABSystem:SimulateUsingDescription
      mask Display:
      | if (strcmp(sysName,'???'))
      | 	color('red');
      | else
      |     color('blue');
      | end
      | text(0.99, 0.99, sysName, 'horizontalAlignment', 'right', 'verticalAlignment','top');
      | 
      | color('black');
      | DescText = ['EE: ' get_param(gcb,'EndEffector')];
      | text(0.5, 0.05, DescText, 'horizontalAlignment', 'center', 'verticalAlignment','bottom');
      | 
      | port_label('input', 1, 'Config')
      | port_label('output', 1, 'Jacobian')
  Terminator : Terminator
  Ja : Outport
  wires:
  Direct Kinematics/1(orientation) -> Analytical from Geometric/2(angles)
  Direct Kinematics/2(position) -> Terminator/1
  Analytical from Geometric/1(Ja) -> Ja/1
  Get Jacobian/1(Jacobian) -> Analytical from Geometric/1(geomJ)
  q/1 -> Get Jacobian/1(Config), Direct Kinematics/1(q)

== system IDC_OS/Trajectory/Direct Kinematics/Get Transform ==
  Config : Inport  PortDimensions=6
  MATLAB System : MATLABSystem  System=robotics.slmanip.internal.block.GetTransformBlock  TreeStruct=TreeStruct  SourceBodyName=SourceBody  TargetBodyName=TargetBody  SimulateUsing=Code generation
      mask Type: robotics.slmanip.internal.block.GetTransformBlock
      mask Display:
      | disp('GetTransformBlock');
      | port_label('input',1,'q');
      | port_label('output',1,'tform');
  Transform : Outport  VectorParamsAs1DForOutWhenUnconnected=off
  wires:
  MATLAB System/1 -> Transform/1
  Config/1 -> MATLAB System/1

== system IDC_OS/Trajectory/Direct Kinematics/extract P and O ==
  In1 : Inport
  Orientation : MATLABFcn  MATLABFcn=tform2rotm  Output1D=off
  Position : MATLABFcn  MATLABFcn=tform2trvec
  orientation : Outport
  position : Outport  Port=2
  wires:
  Orientation/1 -> orientation/1
  In1/1 -> Position/1, Orientation/1
  Position/1 -> position/1

== system IDC_OS/J._A(q,q.)*q./Analytical Jacobian/Direct Kinematics/Get Transform ==
  Config : Inport  PortDimensions=6
  MATLAB System : MATLABSystem  System=robotics.slmanip.internal.block.GetTransformBlock  TreeStruct=TreeStruct  SourceBodyName=SourceBody  TargetBodyName=TargetBody  SimulateUsing=Code generation
      mask Type: robotics.slmanip.internal.block.GetTransformBlock
      mask Display:
      | disp('GetTransformBlock');
      | port_label('input',1,'q');
      | port_label('output',1,'tform');
  Transform : Outport  VectorParamsAs1DForOutWhenUnconnected=off
  wires:
  MATLAB System/1 -> Transform/1
  Config/1 -> MATLAB System/1

== system IDC_OS/J._A(q,q.)*q./Analytical Jacobian/Direct Kinematics/extract P and O ==
  In1 : Inport
  Orientation : MATLABFcn  MATLABFcn=tform2rotm  Output1D=off
  Position : MATLABFcn  MATLABFcn=tform2trvec
  orientation : Outport
  position : Outport  Port=2
  wires:
  Orientation/1 -> orientation/1
  In1/1 -> Position/1, Orientation/1
  Position/1 -> position/1

== system IDC_OS/J_A(q)*q./Analytical Jacobian/Direct Kinematics/Get Transform ==
  Config : Inport  PortDimensions=6
  MATLAB System : MATLABSystem  System=robotics.slmanip.internal.block.GetTransformBlock  TreeStruct=TreeStruct  SourceBodyName=SourceBody  TargetBodyName=TargetBody  SimulateUsing=Code generation
      mask Type: robotics.slmanip.internal.block.GetTransformBlock
      mask Display:
      | disp('GetTransformBlock');
      | port_label('input',1,'q');
      | port_label('output',1,'tform');
  Transform : Outport  VectorParamsAs1DForOutWhenUnconnected=off
  wires:
  MATLAB System/1 -> Transform/1
  Config/1 -> MATLAB System/1

== system IDC_OS/J_A(q)*q./Analytical Jacobian/Direct Kinematics/extract P and O ==
  In1 : Inport
  Orientation : MATLABFcn  MATLABFcn=tform2rotm  Output1D=off
  Position : MATLABFcn  MATLABFcn=tform2trvec
  orientation : Outport
  position : Outport  Port=2
  wires:
  Orientation/1 -> orientation/1
  In1/1 -> Position/1, Orientation/1
  Position/1 -> position/1

== system IDC_OS/J_A^(-1)(q)*[...]/Analytical Jacobian/Direct Kinematics/Get Transform ==
  Config : Inport  PortDimensions=6
  MATLAB System : MATLABSystem  System=robotics.slmanip.internal.block.GetTransformBlock  TreeStruct=TreeStruct  SourceBodyName=SourceBody  TargetBodyName=TargetBody  SimulateUsing=Code generation
      mask Type: robotics.slmanip.internal.block.GetTransformBlock
      mask Display:
      | disp('GetTransformBlock');
      | port_label('input',1,'q');
      | port_label('output',1,'tform');
  Transform : Outport  VectorParamsAs1DForOutWhenUnconnected=off
  wires:
  MATLAB System/1 -> Transform/1
  Config/1 -> MATLAB System/1

== system IDC_OS/J_A^(-1)(q)*[...]/Analytical Jacobian/Direct Kinematics/extract P and O ==
  In1 : Inport
  Orientation : MATLABFcn  MATLABFcn=tform2rotm  Output1D=off
  Position : MATLABFcn  MATLABFcn=tform2trvec
  orientation : Outport
  position : Outport  Port=2
  wires:
  Orientation/1 -> orientation/1
  In1/1 -> Position/1, Orientation/1
  Position/1 -> position/1

== system IDC_OS/Manipulator/J_A^(-1)(q)*[...]/Analytical Jacobian/Direct Kinematics ==
  q : Inport
  Get Transform : Subsystem  mask(Get Transform){RigidBodyTree=robot, SourceBody=tool0, TargetBody=base, SimulateUsing=Code generation}
      mask prompts: RigidBodyTree "robotics:robotslmanip:blockmask:RigidBodyTreePrompt"; SourceBody "robotics:robotslmanip:blockmask:GetTransformSourceBodyPrompt"; TargetBody "robotics:robotslmanip:blockmask:GetTransformTargetBodyPrompt"; SimulateUsing "SystemBlock:MATLABSystem:SimulateUsing"
      mask help: robotics:robotslmanip:blockmask:GetTransformDescription
      mask init: same as IDC_OS/Forward Kinematics K(q)/Direct Kinematics/Get Transform
      settings: LibrarySourceBlock=robotmaniplib/Get Transform
      mask Help: helpview(fullfile(docroot,'robotics','helptargets.map'), 'rstGetTransform');
      mask TypeOptions SimulateUsing: MATLAB System/SimulateUsing
      mask DialogControl RigidBodyTree Prompt: Rigid body tree:
      mask DialogControl SourceBody Prompt: Source body:
      mask DialogControl ListControl1 Prompt: Select body >>
      mask DialogControl ListControl1 Callback: robotics.slmanip.internal.block.RBTAlgorithmBlockMasks.updateMaskBodyList(gcb, 'SourceBody');
      mask DialogControl TargetBody Prompt: Target body:
      mask DialogControl ListControl2 Prompt: Select body >>
      mask DialogControl ListControl2 Callback: robotics.slmanip.internal.block.RBTAlgorithmBlockMasks.updateMaskBodyList(gcb, 'TargetBody');
      mask DialogControl SimulateUsing Prompt: Simulate using:
      mask DialogControl SimulateUsing Tooltip: SystemBlock:MATLABSystem:SimulateUsingDescription
      mask Display:
      | if (strcmp(sysName,'???'))
      | 	color('red');
      | else
      |     color('blue');
      | end
      | text(0.99, 0.99, sysName, 'horizontalAlignment', 'right', 'verticalAlignment','top');
      | 
      | color('black')
      | SourceText = ['Source: ' get_param(gcb,'SourceBody')];
      | TargetText = ['Target: ' get_param(gcb,'TargetBody')];
      | DescText = [SourceText newline TargetText];
      | text(0.5, 0.05, DescText, 'horizontalAlignment', 'center','verticalAlignment','bottom');
      | 
      | port_label('input', 1, 'Config')
      | port_label('output', 1, 'Transform')
  extract P and O : Subsystem
  get RPY angles : MATLAB Function  TreatAsAtomicUnit=on
  orientation : Outport
  position : Outport  Port=2
  wires:
  get RPY angles/1(rpy) -> orientation/1
  extract P and O/1(orientation) -> get RPY angles/1(R)
  extract P and O/2(position) -> position/1
  Get Transform/1(Transform) -> extract P and O/1(In1)
  q/1 -> Get Transform/1(Config)

== system IDC_OS/Manipulator/J_A^(-1)(q)*[...]/Analytical Jacobian/Get Jacobian ==
  Config : Inport  PortDimensions=6
  MATLAB System : MATLABSystem  System=robotics.slmanip.internal.block.GetJacobianBlock  TreeStruct=TreeStruct  EEBodyName=EndEffector  SimulateUsing=Code generation
      mask Type: robotics.slmanip.internal.block.GetJacobianBlock
      mask Display:
      | disp('GetJacobianBlock');
      | port_label('input',1,'q');
      | port_label('output',1,'jacobianMat');
  Jacobian : Outport  VectorParamsAs1DForOutWhenUnconnected=off
  wires:
  MATLAB System/1 -> Jacobian/1
  Config/1 -> MATLAB System/1

== system IDC_OS/Manipulator/J_A^(-1)(q)*[...]/Analytical Jacobian/Direct Kinematics/Get Transform ==
  Config : Inport  PortDimensions=6
  MATLAB System : MATLABSystem  System=robotics.slmanip.internal.block.GetTransformBlock  TreeStruct=TreeStruct  SourceBodyName=SourceBody  TargetBodyName=TargetBody  SimulateUsing=Code generation
      mask Type: robotics.slmanip.internal.block.GetTransformBlock
      mask Display:
      | disp('GetTransformBlock');
      | port_label('input',1,'q');
      | port_label('output',1,'tform');
  Transform : Outport  VectorParamsAs1DForOutWhenUnconnected=off
  wires:
  MATLAB System/1 -> Transform/1
  Config/1 -> MATLAB System/1

== system IDC_OS/Manipulator/J_A^(-1)(q)*[...]/Analytical Jacobian/Direct Kinematics/extract P and O ==
  In1 : Inport
  Orientation : MATLABFcn  MATLABFcn=tform2rotm  Output1D=off
  Position : MATLABFcn  MATLABFcn=tform2trvec
  orientation : Outport
  position : Outport  Port=2
  wires:
  Orientation/1 -> orientation/1
  In1/1 -> Position/1, Orientation/1
  Position/1 -> position/1

== matlab function IDC_OS/Trajectory/Direct Kinematics/get RPY angles ==
  data: R input; rpy output
function rpy = rpyWrap(R)
%rpy = getRPYanglesFromR(R);
[rpy, ~] = eulerInverseProblem(R,'zyx','current');

== matlab function IDC_OS/Manipulator/J_A^(-1)(q)*[...]/inverse ==
  data: u input; y output
function y = fcn(u)

y = pinv(u);
